simulink model "PVArrayGrid100kw"  (R2019a)
settings: Solver=FixedStepDiscrete  StartTime=0.0  StopTime=2.5  RelTol=1e-3
PreLoadFcn:
  | Ts_Power=1e-6;
  | Ts_Control=100e-6;
InitFcn:
  | Ts_Power=1e-6;
  | Ts_Control=100e-6;
undefined symbols (not defined in the file or in its folder): D1, Delta, DiscIntNeverNeededParam
libraries: powerlib x22, powerlib_meascontrol x11, simulink x2, spsGroundingTransformerLib x1, SignalEditorBlockLib x1, re_lib x1
(part 1 of 2)
settings Model: SimulationMode=accelerator  Creator=The MathWorks, Inc.  LastModifiedBy=HP
settings DataIOCC: LimitDataPoints=on  SaveFormat=Array  SignalLogging=off  DSMLogging=off  ReturnWorkspaceOutputs=off
settings OptimizationCC: ExpressionDepthLimit=2147483647  EfficientMapNaN2IntZero=off  LifeSpan=inf
settings DebuggingCC: UnderspecifiedInitializationDetection=Classic  MergeDetectMultiDrivingBlocksExec=none  SolverPrmCheckMsg=warning  FcnCallInpInsideContextMsg=warning  StateNameClashWarn=warning  SFUnexpectedBacktrackingDiag=warning  SFNoUnconditionalDefaultTransitionDiag=warning  SFExecutionAtInitializationDiag=none  ArithmeticOperatorsInVariantConditions=warning
settings HardwareCC: ProdBitPerPointer=32  ProdBitPerSizeT=32  ProdBitPerPtrDiffT=32  ProdLargestAtomicFloat=None  ProdIntDivRoundTo=Undefined  ProdEndianess=Unspecified  ProdWordSize=32  ProdHWDeviceType=32-bit Generic  TargetBitPerPointer=64  TargetBitPerSizeT=64  TargetBitPerPtrDiffT=64  TargetLongLongMode=on  TargetIntDivRoundTo=Zero  TargetEndianess=LittleEndian  TargetWordSize=64  TargetHWDeviceType=MATLAB Host  ProdEqTarget=off
settings ModelReferenceCC: PropagateSignalLabelsOutOfModel=off
settings SFSimCC: SimUseLocalCustomCode=off
settings CodeAppCC: MaxIdLength=128
settings GRTTargetCC: TargetLangStandard=C89/C90 (ANSI)  CombineOutputUpdateFcns=off  GRTInterface=on
settings ConfigComp: CovMetricSettings=dw  CovSaveCumulativeToWorkspaceVar=on  CovSaveSingleToWorkspaceVar=on  CovExternalEMLEnable=off  CovSFcnEnable=off
settings SimscapeCC: SimscapeNormalizeSystem=off

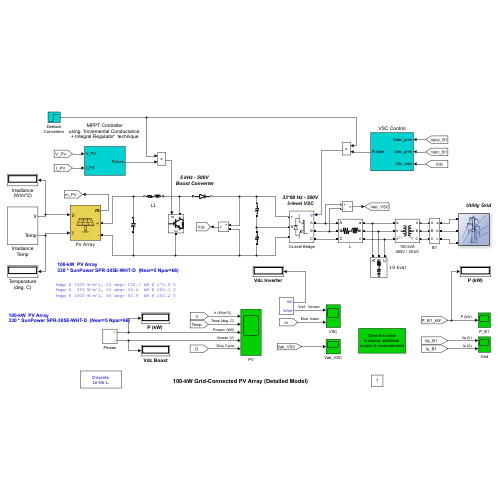
[thumbnail: Simulink's stored preview of the top-level diagram]
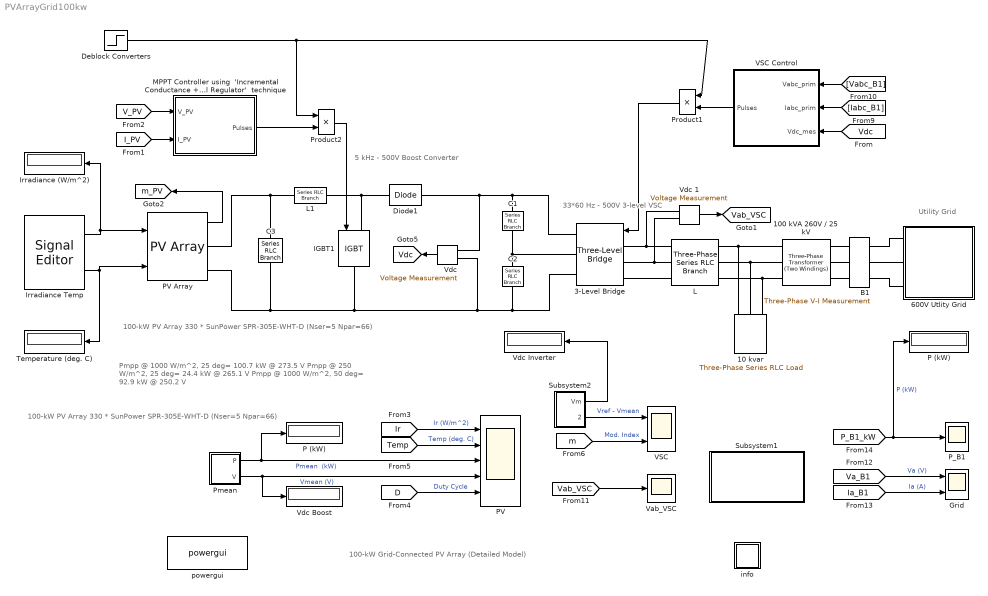
== system PVArrayGrid100kw ==
  note: 5 kHz - 500V
      | Boost Converter
  note: 33*60 Hz - 500V
      | 3-level VSC
  note: 100-kW Grid-Connected PV Array (Detailed Model)
  note: Utility Grid
  note: Pmpp @ 1000 W/m^2, 25 deg= 100.7 kW @ 273.5 V
      | Pmpp @  250 W/m^2, 25 deg= 24.4  kW @ 265.1 V
      | Pmpp @ 1000 W/m^2, 50 deg= 92.9  kW @ 250.2 V
  note: 100-kW  PV Array
      | 330 * SunPower SPR-305E-WHT-D  (Nser=5 Npar=66)
  note: 100-kW  PV Array
      | 330 * SunPower SPR-305E-WHT-D  (Nser=5 Npar=66)
  10 kvar : powerlib/Elements/Three-Phase Series RLC Load  LConnTagsString=A|B|C  Configuration=Y (grounded)  NominalVoltage=240  Vabc=[1e3 1e3 1e3]  Vabcp=[1e3 1e3 1e3]  NominalFrequency=60  UnbalancedPower=off  ActivePower=10e3/100  InductivePower=0  CapacitivePower=10e3  Pabc=[10e3 9e3 11e3]  QLabc=[100 90 110]  QCabc=[100 90 110]  Pabcp=[10e3 9e3 11e3]  QLabcp=[100 90 110]  QCabcp=[100 90 110]  Measurements=None  LoadType=constant Z
  100 kVA 260V / 25 kV : powerlib/Elements/Three-Phase Transformer (Two Windings)  Winding1Connection=Yg  Winding2Connection=Delta (D1)  CoreType=Three single-phase transformers  SetSaturation=off  Hysteresis=off  DataFile='hysteresis'  SetInitialFlux=off  Measurements=None  UNITS=pu  NominalPower=[100e3 , 60 ]  Winding1=[ 25e3 , 0.001 , 0.03 ]  Winding2=[ 260 , 0.001 , 0.03 ]  Rm=500  Lm=500  L0=0.5  Saturation=[ 0,0 ; 0.0024,1.2 ; 1.0,1.52 ]  InitialFluxes=[ 0.8 , -0.8 , 0.7 ]  BreakLoop=off  DiscreteSolver=Trapezoidal iterative  DataType=off  TransfoNumber=0
  3-Level Bridge : powerlib/Power Electronics/Three-Level Bridge  Arms=3  SnubberResistance=1e6  SbubberCapacitance=inf  Device=IGBT / Diodes  Ron=0.2e-3  ForwardVoltages="[  0  0 ]"  Measurements=None
  600V Utlity Grid : Subsystem
      mask Display: image('grid.jpg')
  B1 : powerlib/Measurements/Three-Phase V-I Measurement  VoltageMeasurement=phase-to-ground  SetLabelV=on  LabelV=Vabc_B1  Vpu=off  VpuLL=off  CurrentMeasurement=yes  SetLabelI=on  LabelI=Iabc_B1  Ipu=off  Pbase=100e6  Vbase=500e3  OutputType=Magnitude  PhasorSimulation=off  PSBequivalent=0
  C1 : powerlib/Elements/Series RLC Branch  LConnTagsString=__new0  RConnTagsString=__new0  BranchType=C  Resistance=1.0  Inductance=1.0  SetiL0=off  InitialCurrent=0  Capacitance=12000e-06  Setx0=off  InitialVoltage=0  Measurements=None
  C2 : powerlib/Elements/Series RLC Branch  LConnTagsString=__new0  RConnTagsString=__new0  BranchType=C  Resistance=1.0  Inductance=1.0  SetiL0=off  InitialCurrent=0  Capacitance=12000e-06  Setx0=off  InitialVoltage=0  Measurements=None
  C3 : powerlib/Elements/Series RLC Branch  LConnTagsString=__new0  RConnTagsString=__new0  BranchType=C  Resistance=1.0  Inductance=1.0  SetiL0=off  InitialCurrent=0  Capacitance=100e-6  Setx0=off  InitialVoltage=0  Measurements=Branch voltage
  Deblock Converters : Step  Time=0.05  SampleTime=0
  Diode1 : powerlib/Power Electronics/Diode  Ron=1e-4  Lon=0  Vf=0  IC=0  UseSnubber=off  Rs=inf  Cs=inf  Measurements=off
  Grid : Scope  NumInputPorts=2
  IGBT1 : powerlib/Power Electronics/IGBT  Ron=0.001  Lon=0  Vf=0  Tf=0  Tt=0  IC=0  Rs=1e5  Cs=inf  Measurements=off
  Irradiance (W/m^2) : Display
      settings: Format=bank  Decimation=1000
  Irradiance Temp : SignalEditorBlockLib/Signal Editor  FileName=PVArrayGridData.mat  ActiveScenario=Ramp_up_down_Irradiance  ActiveSignal=Temp  IsBus=off  OutputBusObjectStr=Bus: BusObject  SampleTime=0  OutputAfterFinalValue=Extrapolation  Unit=inherit  PreserveSignalName=on
  L : powerlib/Elements/Three-Phase Series RLC Branch  LConnTagsString=A|B|C  RConnTagsString=A|B|C  BranchType=RL  Resistance=500e-6*377/50/2  Inductance=500e-6/2  Capacitance=inf  Measurements=None
  L1 : powerlib/Elements/Series RLC Branch  LConnTagsString=__new0  RConnTagsString=__new0  BranchType=RL  Resistance=0.005  Inductance=5e-3  SetiL0=off  InitialCurrent=0  Capacitance=1e-6  Setx0=off  InitialVoltage=0  Measurements=None
  "MPPT Controller using  'Incremental Conductance + Integral Regulator'  technique " : Subsystem  mask(Boost Control - MPPT){fc=5000, T_MPPT=200e-6, Dinit=0.5}
      mask prompts: fc "PWM switching frequency (Hz)"; T_MPPT "Time window used by MPPT control (s)"; Dinit "Initial value of duty cycle"
  P (kW) : Display
      settings: Format=bank  Decimation=2000
  "P (kW) " : Display
      settings: Format=bank  Decimation=2000
  PV : Scope  NumInputPorts=5
  PV Array : re_lib/Solar/PV Array  Npar=66  Nser=5  PlotType=array @ 1000 W/m2 & specified temperatures  S_vec="[ 1000  250 ]"  Temp_C_vec="[0 25 50  ]"  ModuleName=SunPower SPR-305E-WHT-D  PlotWhenSelected=off  Pm=305.226  Ncell=96  Voc=64.2  Isc=5.96  Vm=54.7  Im=5.58  beta_Voc_pc=-0.2727  alpha_Isc_pc=0.061745  beta_Voc=-0.17507  alpha_Isc=0.00368  IL=5.9657  I0=6.3076e-12  nI=0.94489  Rsh=393.2054  Rs=0.37428  RobustModel=off  RobustCellTemperature=25  BAL=on  Tc=1e-6  Tfilter=5e-5
  P_B1 : Scope
  Pmean : Subsystem
  Product1 : Product  RndMeth=Zero
  Product2 : Product  RndMeth=Zero
  Subsystem1 : Subsystem
      mask Display: disp('Open this block\nto display additional \nscopes & measurements')
  Subsystem2 : Subsystem
  Temperature (deg. C) : Display
      settings: Format=bank  Decimation=1000
  VSC : Scope  NumInputPorts=2
  VSC Control : Subsystem  mask(VSC Main Controller){nom=[ 100e3  60 ], Vnom=[ 25e3 260 ], Vnom_dc=500, RLxfo=[0.002  0.06 ], RLchoke=[2e-3  250e-6  ], K_VDCreg=[7  800], K_Ireg=[0.3 20], Ts=Ts_Control}
      mask prompts: nom "Nominal power and frequency [ Pnom(VA)  Fnom(Hz) ]:"; Vnom "Nominal primary and secondary voltages (Vrms LL) [ Vnom_prim   Vnom_sec ]:"; Vnom_dc "Nominal DC bus voltage (V):"; RLxfo "Total transformer leakage impedance (pu/Pnom) [ Rxfo  Lxf ]"; RLchoke "Choke impedance [ R(ohm) L(H) ]"; K_VDCreg "VDC regultator gains [ Kp  Ki ]:"; K_Ireg "Current regulator gains [ Kp  Ki ]:"; Ts "Sample time"
      mask init:
      | Pnom=nom(1);
      | Fnom=nom(2);
      | Vnom_prim=Vnom(1);
      | Vnom_sec=Vnom(2);
      | Zbase=Vnom_sec^2/Pnom;
      | Rtot_pu=RLxfo(1) + RLchoke(1)/Zbase;
      | Ltot_pu=RLxfo(2) + RLchoke(2)/(Zbase/(2*pi*Fnom));
      | Kp_VDCreg=K_VDCreg(1);
      | Ki_VDCreg=K_VDCreg(2);
      | Kp_Ireg=K_Ireg(1);
      | Ki_Ireg=K_Ireg(2);
      | Vdc_ref=Vnom_dc;
      | % Used to determine initial value of Boost Control (MPPT)
      | assignin('base','Vdc_ref_Inv',Vdc_ref);
  Vab_VSC : Scope
  "Vdc " : powerlib/Measurements/Voltage Measurement  Tag=PoWeRsYsTeMmEaSuReMeNt  PhasorSimulation=off  OutputType=Magnitude  PSBequivalent=0
  Vdc 1 : powerlib/Measurements/Voltage Measurement  Tag=PoWeRsYsTeMmEaSuReMeNt  PhasorSimulation=off  OutputType=Magnitude  PSBequivalent=0
  Vdc Boost : Display
      settings: Format=bank  Decimation=2000
  Vdc Inverter : Display
      settings: Format=bank  Decimation=2000
  info : Subsystem
      settings: OpenFcn="showExample(\"simscapeelectricalsps/PVArrayGridExample\")"
      mask Display: disp('?')
  powergui : powerlib/powergui  Priority=1  SimulationMode=Discrete  SampleTime=Ts_Power  frequency=60  Iterations=50  frequencyindice=0  Pbase=100e6  ErrMax=1e-4  UnitsV=kV  UnitsW=MW  buscounter=0  FunctionMessages=off  echomessages=off  EnableUseOfTLC=off  CurrentSourceSwitches=off  DisableSnubberDevices=off  DisableRonSwitches=off  DisableVfSwitches=off  DisplayEquations=off  AutomaticDiscreteSolvers=off  SolverType=Tustin/Backward Euler (TBE)  Interpol=off  ExternalGateDelay=off  methode=off  Ts=0  x0status=blocks  SPID=off  SwTol=0  HookPort=off  NonlinearTolerance=1e-8  nMaxIteration=10  ContinueOnMaxIteration=off  RestoreLinks=warning  ResistiveCurrentMeasurement=off  Frange=[0:2:500]  Ylog=off  Xlog=on  ShowGrid=off  save=off  variable=ZData  structure=0  ZoomFFT=on  StartTime=0.0  cycles=1  DisplayStyle=1  fundamental=60  FreqAxis=off  MaxFrequency=1000  frequencyindicesteady=1  RmsSteady=1  display=off
  tag scope: Vab_VSC=global, Vdc=global, m_PV=global
  wires:
  "Vdc "/1 -> [Vdc]
  Product2/1 -> IGBT1/1
  "MPPT Controller using  'Incremental Conductance + Integral Regulator'  technique "/1(Pulses) -> Product2/2
  Deblock Converters/1 -> Product1/1, Product2/1
  [Vabc_B1] -> VSC Control/1(Vabc_prim)
  [Iabc_B1] -> VSC Control/2(Iabc_prim)
  [Vdc] -> VSC Control/3(Vdc_mes)
  VSC Control/1(Pulses) -> Product1/2
  Product1/1 -> 3-Level Bridge/1
  [I_PV] -> "MPPT Controller using  'Incremental Conductance + Integral Regulator'  technique "/2(I_PV)
  [V_PV] -> "MPPT Controller using  'Incremental Conductance + Integral Regulator'  technique "/1(V_PV)
  Pmean/1(P) -> "P (kW) "/1, PV/3  "Pmean  (kW)"
  [m] -> VSC/2  "Mod. Index"
  Vdc 1/1 -> [Vab_VSC]
  [Vab_VSC] -> Vab_VSC/1
  [Ia_B1] -> Grid/2  "Ia (A)"
  [Va_B1] -> Grid/1  "Va (V)"
  [P_B1_kW] -> P_B1/1, P (kW)/1  "P (kW)"
  Pmean/2(V) -> Vdc Boost/1, PV/4  "Vmean (V)"
  Subsystem2/2(VrVm) -> VSC/1  "Vref - Vmean"
  Subsystem2/1(Vm) -> Vdc Inverter/1
  PV Array/1 -> [m_PV]
  Irradiance Temp/1 -> PV Array/1, Irradiance (W/m^2)/1
  Irradiance Temp/2 -> PV Array/2, Temperature (deg. C)/1
  [D] -> PV/5  "Duty Cycle"
  [Temp] -> PV/2  "Temp (deg. C)"
  [Ir] -> PV/1  "Ir (W/m^2)"
  connections:
  3-Level Bridge/RConn1 -- Diode1/RConn1 -- "Vdc "/LConn1 -- C1/LConn1
  L1/RConn1 -- Diode1/LConn1 -- IGBT1/LConn1
  3-Level Bridge/RConn3 -- C2/RConn1 -- "Vdc "/LConn2 -- IGBT1/RConn1 -- PV Array/RConn2 -- C3/RConn1
  3-Level Bridge/LConn1 -- L/LConn1 -- Vdc 1/LConn1
  3-Level Bridge/LConn2 -- L/LConn2 -- Vdc 1/LConn2
  3-Level Bridge/LConn3 -- L/LConn3
  L/RConn1 -- 100 kVA 260V / 25 kV/RConn1 -- 10 kvar/LConn1
  L/RConn2 -- 100 kVA 260V / 25 kV/RConn2 -- 10 kvar/LConn2
  L/RConn3 -- 100 kVA 260V / 25 kV/RConn3 -- 10 kvar/LConn3
  B1/LConn1 -- 100 kVA 260V / 25 kV/LConn1
  B1/LConn2 -- 100 kVA 260V / 25 kV/LConn2
  B1/LConn3 -- 100 kVA 260V / 25 kV/LConn3
  C2/LConn1 -- C1/RConn1 -- 3-Level Bridge/RConn2
  C3/LConn1 -- PV Array/RConn1 -- L1/LConn1
  B1/RConn2 -- 600V Utlity Grid/LConn2
  B1/RConn1 -- 600V Utlity Grid/LConn1
  B1/RConn3 -- 600V Utlity Grid/LConn3

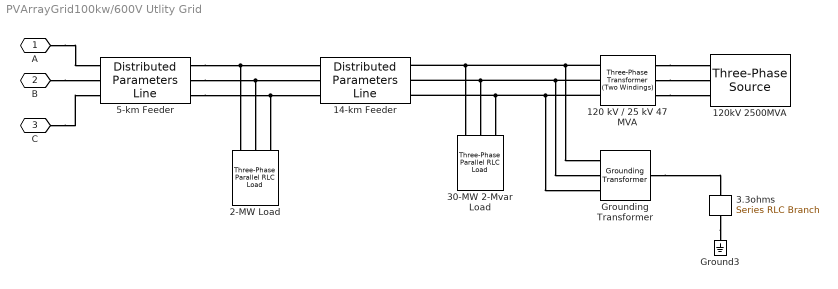
== system PVArrayGrid100kw/600V Utlity Grid ==
  120 kV / 25 kV 47 MVA : powerlib/Elements/Three-Phase Transformer (Two Windings)  Winding1Connection=Yg  Winding2Connection=Delta (D1)  CoreType=Three single-phase transformers  SetSaturation=off  Hysteresis=off  DataFile='basic_model'  SetInitialFlux=off  Measurements=None  UNITS=pu  NominalPower=[47e6 60 ]  Winding1="[ 120e3  0.08/30   0.08 ]"  Winding2="[ 25e3  0.08/30  0.08]"  Rm=500  Lm=500  L0=0.5  Saturation="[ 0,0  ;  0.005,1.2  ;  1.0,1.4 ]"  InitialFluxes=[ 0.8 , -0.8 , 0.7 ]  BreakLoop=off  DiscreteSolver=Trapezoidal iterative  DataType=off  TransfoNumber=0
  120kV 2500MVA : powerlib/Electrical Sources/Three-Phase Source  InternalConnection=Yg  VoltagePhases=off  Voltage=120e3  PhaseAngle=0  Voltage_phases=[25e3 25e3 25e3]/sqrt(3)  PhaseAngles_phases=[0 -120 +120]  Frequency=60  NonIdealSource=on  SpecifyImpedance=on  Resistance=0.8929  Inductance=16.58e-3  ShortCircuitLevel=2500e6  BaseVoltage=120e3  XRratio=7  BusType=swing  Pref=0  Qref=0  Prefabc=[10e3, 10e3, 10e3]  Qrefabc=[0, 0, 0]  Qmin=-inf  Qmax=inf
  14-km Feeder : powerlib/Elements/Distributed Parameters Line  Phases=3  Length=14  Frequency=60  Resistance=[0.1153 0.413]  Inductance=[1.05e-3 3.32e-3]  Capacitance=[11.33e-009 5.01e-009]  x1=[-5.8e-05 -3.04262372149305e-09 0 0;-5.7e-05 -3.04220635150541e-09 0 0;-5.6e-05 -3.0417885491524e-09 0 0;-5.5e-05 -3.04137031449339e-09 0 0;-5.4e-05 -3.04095164758784e-09 0 0;-5.3e-05 -3.04053254849524e-09 0 0;-5.2e-05 -3.04011301727516e-09 0 0;-5.1e-05 -3.03969305398722e-09 0 0;-5e-05 -3.0392726586911e-09 0 0;-4.9e-05 -3.03885183144656e-09 -3790.73535189758 -24061.413420025;-4.8e-05 -3.0384305723134e-09 -3781.66414358218 -24062.8407837194;-4.7e-05 -3.0380088813515e-09 -3772.59239780798 -24064.2647275475;-4.6e-05 -3.03758675862078e-09 -3763.52011586425 -24065.6852513069;-4.5e-05 -3.03716420418123e-09 -3754.44729904039 -24067.1023547957;-4.4e-05 -3.03674121809293e-09 -3745.37394862584 -24068.5160378125;-4.3e-05 -3.03631780041596e-09 -3736.30006591012 -24069.9263001565;-4.2e-05 -3.03589395121053e-09 -3727.22565218283 -24071.3331416271;-4.1e-05 -3.03546967053686e-09 -3718.15070873366 -24072.7365620244;-4e-05 -3.03504495845525e-09 -3709.07523685234 -24074.136561149;-3.9e-05 -3.03461981502607e-09 -3699.99923782872 -24075.5331388019;-3.8e-05 -3.03419424030973e-09 -3690.92271295269 -24076.9262947847;-3.7e-05 -3.03376823436673e-09 -3681.84566351423 -24078.3160288992;-3.6e-05 -3.0333417972576e-09 -3672.76809080339 -24079.7023409481;-3.5e-05 -3.03291492904295e-09 -3663.6899961103 -24081.0852307342;-3.4e-05 -3.03248762978346e-09 -3654.61138072515 -24082.4646980611;-3.3e-05 -3.03205989953984e-09 -3645.53224593822 -24083.8407427326;-3.2e-05 -3.03163173837289e-09 -3636.45259303985 -24085.2133645533;-3.1e-05 -3.03120314634346e-09 -3627.37242332047 -24086.582563328;-3e-05 -3.03077412351246e-09 -3618.29173807058 -24087.9483388622;-2.9e-05 -3.03034466994086e-09 -3609.21053858073 -24089.3106909617;-2.8e-05 -3.02991478568971e-09 -3600.12882614158 -24090.6696194329;-2.7e-05 -3.02948447082009e-09 -3591.04660204383 -24092.0251240827;-2.6e-05 -3.02905372539317e-09 -3581.96386757827 -24093.3772047185;-2.5e-05 -3.02862254947016e-09 -3572.88062403576 -24094.725861148;-2.4e-05 -3.02819094311234e-09 -3563.79687270724 -24096.0710931796;-2.3e-05 -3.02775890638106e-09 -3554.7126148837 -24097.4129006222;-2.2e-05 -3.02732643933771e-09 -3545.62785185622 -24098.7512832849;-2.1e-05 -3.02689354204376e-09 -3536.54258491595 -24100.0862409777;-2e-05 -3.02646021456073e-09 -3527.4568153541 -24101.4177735107;-1.9e-05 -3.02602645695021e-09 -3518.37054446198 -24102.7458806947;-1.8e-05 -3.02559226927385e-09 -3509.28377353094 -24104.0705623411;-1.7e-05 -3.02515765159334e-09 -3500.19650385241 -24105.3918182614;-1.6e-05 -3.02472260397047e-09 -3491.10873671789 -24106.709648268;-1.5e-05 -3.02428712646707e-09 -3482.02047341897 -24108.0240521735;-1.4e-05 -3.02385121914501e-09 -3472.93171524728 -24109.3350297912;-1.3e-05 -3.02341488206626e-09 -3463.84246349454 -24110.6425809346;-1.2e-05 -3.02297811529282e-09 -3454.75271945254 -24111.9467054181;-1.1e-05 -3.02254091888678e-09 -3445.66248441313 -24113.2474030561;-1e-05 -3.02210329291027e-09 -3436.57175966824 -24114.544673664;-9e-06 -3.02166523742548e-09 -3427.48054650986 -24115.8385170573;-8e-06 -3.02122675249467e-09 -3418.38884623006 -24117.128933052;-7e-06 -3.02078783818016e-09 -3409.29666012096 -24118.4159214649;-6e-06 -3.02034849454434e-09 -3400.20398947478 -24119.6994821131;-5e-06 -3.01990872164963e-09 -3391.11083558378 -24120.979614814;-4e-06 -3.01946851955854e-09 -3382.0171997403 -24122.2563193858;-3e-06 -3.01902788833364e-09 -3372.92308323675 -24123.529595647;-2e-06 -3.01858682803754e-09 -3363.82848736561 -24124.7994434166;-1e-06 -3.01814533873294e-09 -3354.73341341942 -24126.0658625142]  x2=[-5.8e-05 -3.19786387480592e-09 0 0;-5.7e-05 -3.19737360997783e-09 0 0;-5.6e-05 -3.19688289073164e-09 0 0;-5.5e-05 -3.1963917171371e-09 0 0;-5.4e-05 -3.19590008926401e-09 0 0;-5.3e-05 -3.19540800718224e-09 0 0;-5.2e-05 -3.19491547096173e-09 0 0;-5.1e-05 -3.19442248067248e-09 0 0;-5e-05 -3.19392903638456e-09 0 0;-4.9e-05 -3.19343513816809e-09 -3379.39242591108 -24244.0512732151;-4.8e-05 -3.19294078609326e-09 -3370.25239397928 -24245.323551305;-4.7e-05 -3.19244598023035e-09 -3361.11188305944 -24246.5923835937;-4.6e-05 -3.19195072064966e-09 -3351.97089445066 -24247.8577699009;-4.5e-05 -3.19145500742159e-09 -3342.82942945205 -24249.1197100467;-4.4e-05 -3.19095884061659e-09 -3333.68748936283 -24250.3782038519;-4.3e-05 -3.19046222030517e-09 -3324.54507548227 -24251.6332511374;-4.2e-05 -3.18996514655792e-09 -3315.40218910971 -24252.884851725;-4.1e-05 -3.18946761944548e-09 -3306.25883154457 -24254.1330054368;-4e-05 -3.18896963903856e-09 -3297.1150040863 -24255.3777120954;-3.9e-05 -3.18847120540794e-09 -3287.97070803447 -24256.6189715239;-3.8e-05 -3.18797231862445e-09 -3278.82594468867 -24257.8567835459;-3.7e-05 -3.18747297875899e-09 -3269.68071534858 -24259.0911479854;-3.6e-05 -3.18697318588254e-09 -3260.53502131394 -24260.3220646671;-3.5e-05 -3.18647294006612e-09 -3251.38886388456 -24261.5495334159;-3.4e-05 -3.18597224138084e-09 -3242.24224436031 -24262.7735540575;-3.3e-05 -3.18547108989785e-09 -3233.09516404113 -24263.9941264179;-3.2e-05 -3.18496948568837e-09 -3223.94762422702 -24265.2112503236;-3.1e-05 -3.1844674288237e-09 -3214.79962621805 -24266.4249256016;-3e-05 -3.18396491937519e-09 -3205.65117131437 -24267.6351520794;-2.9e-05 -3.18346195741426e-09 -3196.50226081616 -24268.841929585;-2.8e-05 -3.18295854301239e-09 -3187.35289602369 -24270.045257947;-2.7e-05 -3.18245467624112e-09 -3178.20307823729 -24271.2451369943;-2.6e-05 -3.18195035717207e-09 -3169.05280875736 -24272.4415665564;-2.5e-05 -3.18144558587691e-09 -3159.90208888434 -24273.6345464632;-2.4e-05 -3.18094036242738e-09 -3150.75091991877 -24274.8240765452;-2.3e-05 -3.18043468689528e-09 -3141.59930316123 -24276.0101566333;-2.2e-05 -3.17992855935249e-09 -3132.44723991236 -24277.192786559;-2.1e-05 -3.17942197987093e-09 -3123.29473147288 -24278.3719661542;-2e-05 -3.1789149485226e-09 -3114.14177914356 -24279.5476952513;-1.9e-05 -3.17840746537956e-09 -3104.98838422525 -24280.7199736831;-1.8e-05 -3.17789953051394e-09 -3095.83454801884 -24281.8888012832;-1.7e-05 -3.17739114399792e-09 -3086.68027182529 -24283.0541778853;-1.6e-05 -3.17688230590375e-09 -3077.52555694565 -24284.2161033239;-1.5e-05 -3.17637301630377e-09 -3068.37040468099 -24285.3745774338;-1.4e-05 -3.17586327527034e-09 -3059.21481633246 -24286.5296000503;-1.3e-05 -3.17535308287591e-09 -3050.05879320128 -24287.6811710094;-1.2e-05 -3.17484243919299e-09 -3040.90233658873 -24288.8292901473;-1.1e-05 -3.17433134429415e-09 -3031.74544779614 -24289.9739573009;-1e-05 -3.17381979825204e-09 -3022.5881281249 -24291.1151723075;-9e-06 -3.17330780113935e-09 -3013.43037887649 -24292.2529350049;-8e-06 -3.17279535302886e-09 -3004.27220135241 -24293.3872452314;-7e-06 -3.17228245399339e-09 -2995.11359685425 -24294.5181028257;-6e-06 -3.17176910410583e-09 -2985.95456668366 -24295.6455076273;-5e-06 -3.17125530343915e-09 -2976.79511214232 -24296.7694594758;-4e-06 -3.17074105206636e-09 -2967.63523453202 -24297.8899582115;-3e-06 -3.17022635006056e-09 -2958.47493515457 -24299.0070036751;-2e-06 -3.16971119749489e-09 -2949.31421531184 -24300.1205957079;-1e-06 -3.16919559444257e-09 -2940.1530763058 -24301.2307341517]  x3=[-5.8e-05 -1.60560160529195e-11 0 0;-5.7e-05 -1.60568474458934e-11 0 0;-5.6e-05 -1.60576765568311e-11 0 0;-5.5e-05 -1.6058503385615e-11 0 0;-5.4e-05 -1.60593279321273e-11 0 0;-5.3e-05 -1.60601501962511e-11 0 0;-5.2e-05 -1.60609701778693e-11 0 0;-5.1e-05 -1.60617878768654e-11 0 0;-5e-05 -1.60626032931233e-11 0 0;-4.9e-05 -1.60634164265271e-11 -23.5442847382492 -155.681477773822;-4.8e-05 -1.60642272769611e-11 -23.4855925321305 -155.690342696943;-4.7e-05 -1.60650358443102e-11 -23.4268969881853 -155.699185492994;-4.6e-05 -1.60658421284594e-11 -23.3681981147557 -155.708006160718;-4.5e-05 -1.60666461292941e-11 -23.3094959201839 -155.716804698862;-4.4e-05 -1.60674478467001e-11 -23.2507904128129 -155.725581106176;-4.3e-05 -1.60682472805634e-11 -23.1920816009861 -155.734335381411;-4.2e-05 -1.60690444307705e-11 -23.1333694930472 -155.743067523325;-4.1e-05 -1.6069839297208e-11 -23.0746540973407 -155.751777530675;-4e-05 -1.60706318797629e-11 -23.0159354222111 -155.760465402224;-3.9e-05 -1.60714221783226e-11 -22.9572134760039 -155.769131136737;-3.8e-05 -1.60722101927748e-11 -22.8984882670646 -155.777774732983;-3.7e-05 -1.60729959230076e-11 -22.8397598037395 -155.786396189732;-3.6e-05 -1.60737793689091e-11 -22.7810280943752 -155.794995505761;-3.5e-05 -1.60745605303681e-11 -22.7222931473187 -155.803572679846;-3.4e-05 -1.60753394072736e-11 -22.6635549709176 -155.812127710769;-3.3e-05 -1.60761159995148e-11 -22.6048135735199 -155.820660597314;-3.2e-05 -1.60768903069815e-11 -22.5460689634741 -155.829171338267;-3.1e-05 -1.60776623295634e-11 -22.487321149129 -155.83765993242;-3e-05 -1.6078432067151e-11 -22.4285701388341 -155.846126378567;-2.9e-05 -1.60791995196349e-11 -22.3698159409392 -155.854570675503;-2.8e-05 -1.60799646869058e-11 -22.3110585637946 -155.862992822028;-2.7e-05 -1.60807275688552e-11 -22.252298015751 -155.871392816947;-2.6e-05 -1.60814881653746e-11 -22.1935343051596 -155.879770659064;-2.5e-05 -1.60822464763559e-11 -22.134767440372 -155.88812634719;-2.4e-05 -1.60830025016912e-11 -22.0759974297402 -155.896459880136;-2.3e-05 -1.60837562412733e-11 -22.017224281617 -155.904771256719;-2.2e-05 -1.60845076949949e-11 -21.9584480043551 -155.913060475756;-2.1e-05 -1.60852568627492e-11 -21.8996686063081 -155.921327536071;-2e-05 -1.60860037444298e-11 -21.8408860958297 -155.929572436487;-1.9e-05 -1.60867483399305e-11 -21.7821004812744 -155.937795175834;-1.8e-05 -1.60874906491456e-11 -21.7233117709968 -155.945995752943;-1.7e-05 -1.60882306719694e-11 -21.6645199733521 -155.954174166647;-1.6e-05 -1.60889684082968e-11 -21.605725096696 -155.962330415786;-1.5e-05 -1.60897038580231e-11 -21.5469271493845 -155.970464499199;-1.4e-05 -1.60904370210435e-11 -21.4881261397741 -155.978576415731;-1.3e-05 -1.60911678972541e-11 -21.4293220762218 -155.986666164228;-1.2e-05 -1.60918964865508e-11 -21.3705149670848 -155.994733743541;-1.1e-05 -1.60926227888302e-11 -21.3117048207212 -156.002779152524;-1e-05 -1.60933468039889e-11 -21.2528916454889 -156.010802390033;-9e-06 -1.60940685319242e-11 -21.1940754497468 -156.018803454927;-8e-06 -1.60947879725334e-11 -21.135256241854 -156.02678234607;-7e-06 -1.60955051257143e-11 -21.0764340301698 -156.034739062328;-6e-06 -1.6096219991365e-11 -21.0176088230543 -156.042673602569;-5e-06 -1.60969325693838e-11 -20.9587806288679 -156.050585965666;-4e-06 -1.60976428596695e-11 -20.8999494559714 -156.058476150495;-3e-06 -1.60983508621212e-11 -20.8411153127259 -156.066344155934;-2e-06 -1.60990565766382e-11 -20.7822782074932 -156.074189980865;-1e-06 -1.60997600031202e-11 -20.7234381486352 -156.082013624173]  x4=[-5.8e-05 7.96597166434352e-12 0 0;-5.7e-05 7.96849067585659e-12 0 0;-5.6e-05 7.97100855486942e-12 0 0;-5.5e-05 7.97352530102418e-12 0 0;-5.4e-05 7.97604091396316e-12 0 0;-5.3e-05 7.97855539332885e-12 0 0;-5.2e-05 7.98106873876388e-12 0 0;-5.1e-05 7.98358094991106e-12 0 0;-5e-05 7.98609202641334e-12 0 0;-4.9e-05 7.98860196791383e-12 -1.35581366009424 -2.15298522698338;-4.8e-05 7.99111077405583e-12 -1.3550019074591 -2.15349620368578;-4.7e-05 7.99361844448276e-12 -1.35418996224797 -2.15400687432833;-4.6e-05 7.99612497883825e-12 -1.35337782457625 -2.15451723883847;-4.5e-05 7.99863037676605e-12 -1.35256549455936 -2.15502729714366;-4.4e-05 8.0011346379101e-12 -1.35175297231274 -2.15553704917141;-4.3e-05 8.00363776191446e-12 -1.35094025795188 -2.15604649484927;-4.2e-05 8.00613974842341e-12 -1.35012735159228 -2.15655563410485;-4.1e-05 8.00864059708135e-12 -1.34931425334948 -2.15706446686577;-4e-05 8.01114030753286e-12 -1.34850096333903 -2.15757299305973;-3.9e-05 8.01363887942267e-12 -1.34768748167652 -2.15808121261444;-3.8e-05 8.01613631239567e-12 -1.34687380847756 -2.15858912545769;-3.7e-05 8.01863260609693e-12 -1.34605994385779 -2.15909673151728;-3.6e-05 8.02112776017167e-12 -1.34524588793289 -2.15960403072108;-3.5e-05 8.02362177426527e-12 -1.34443164081854 -2.16011102299698;-3.4e-05 8.02611464802327e-12 -1.34361720263048 -2.16061770827293;-3.3e-05 8.02860638109139e-12 -1.34280257348445 -2.16112408647691;-3.2e-05 8.03109697311548e-12 -1.34198775349622 -2.16163015753697;-3.1e-05 8.0335864237416e-12 -1.34117274278161 -2.16213592138118;-3e-05 8.03607473261591e-12 -1.34035754145644 -2.16264137793765;-2.9e-05 8.03856189938479e-12 -1.33954214963657 -2.16314652713455;-2.8e-05 8.04104792369475e-12 -1.33872656743788 -2.16365136890008;-2.7e-05 8.04353280519248e-12 -1.3379107949763 -2.16415590316251;-2.6e-05 8.0460165435248e-12 -1.33709483236775 -2.16466012985012;-2.5e-05 8.04849913833874e-12 -1.33627867972821 -2.16516404889124;-2.4e-05 8.05098058928145e-12 -1.33546233717367 -2.16566766021427;-2.3e-05 8.05346089600027e-12 -1.33464580482014 -2.16617096374763;-2.2e-05 8.05594005814269e-12 -1.33382908278368 -2.16667395941978;-2.1e-05 8.05841807535637e-12 -1.33301217118037 -2.16717664715924;-2e-05 8.06089494728912e-12 -1.33219507012629 -2.16767902689457;-1.9e-05 8.06337067358893e-12 -1.33137777973759 -2.16818109855437;-1.8e-05 8.06584525390394e-12 -1.33056030013041 -2.16868286206727;-1.7e-05 8.06831868788246e-12 -1.32974263142094 -2.16918431736198;-1.6e-05 8.07079097517295e-12 -1.32892477372538 -2.16968546436722;-1.5e-05 8.07326211542406e-12 -1.32810672715998 -2.17018630301177;-1.4e-05 8.07573210828457e-12 -1.32728849184099 -2.17068683322444;-1.3e-05 8.07820095340344e-12 -1.32647006788471 -2.17118705493411;-1.2e-05 8.08066865042981e-12 -1.32565145540744 -2.17168696806968;-1.1e-05 8.08313519901294e-12 -1.32483265452554 -2.17218657256009;-1e-05 8.0856005988023e-12 -1.32401366535538 -2.17268586833435;-9e-06 8.08806484944748e-12 -1.32319448801335 -2.17318485532149;-8e-06 8.09052795059828e-12 -1.32237512261586 -2.1736835334506;-7e-06 8.09298990190462e-12 -1.32155556927939 -2.1741819026508;-6e-06 8.09545070301661e-12 -1.32073582812039 -2.17467996285127;-5e-06 8.09791035358451e-12 -1.31991589925538 -2.17517771398121;-4e-06 8.10036885325875e-12 -1.31909578280088 -2.17567515596989;-3e-06 8.10282620168993e-12 -1.31827547887346 -2.17617228874661;-2e-06 8.1052823985288e-12 -1.31745498758968 -2.17666911224072;-1e-06 8.10773744342627e-12 -1.31663430906618 -2.1771656263816]  x5=5.70973484498186e-05  V1=[0 0 0 2.868e-09 2.436e+04 2.436e+04;0 0 0 377 377 377;1.571 1.571 1.571 -0.5389 -0.156 -1.727]  V2=[0 0 0 2.996e-09 2.448e+04 2.448e+04;0 0 0 377 377 377;1.571 1.571 1.571 -0.5232 -0.1382 -1.709]  I1=[0 0 0 1.022e-11 157.5 157.5;0 0 0 377 377 377;1.571 1.571 1.571 -1.198 -0.1498 -1.721]  I2=[0 0 0 6.231e-12 2.544 2.544;0 0 0 377 377 377;1.571 1.571 1.571 1.184 -0.5617 -2.133]  nHarmo=2  Measurements=None  Decoupling=off  VsMag0=0  VrMag0=0  VsAngle0=0  VrAngle0=0  IsMag0=0  IrMag0=0  IsAngle0=0  IrAngle0=0
  2-MW Load : powerlib/Elements/Three-Phase Parallel RLC Load  LConnTagsString=A|B|C  Configuration=Y (grounded)  NominalVoltage=25e3  Vabc=[1e3 1e3 1e3]  Vabcp=[1e3 1e3 1e3]  NominalFrequency=60  UnbalancedPower=off  ActivePower=2e6  InductivePower=0  CapacitivePower=0  Pabc=[10e3 9e3 11e3]  QLabc=[100 90 110]  QCabc=[100 90 110]  Pabcp=[10e3 9e3 11e3]  QLabcp=[100 90 110]  QCabcp=[100 90 110]  Measurements=None  LoadType=constant Z
  "3.3ohms " : powerlib/Elements/Series RLC Branch  LConnTagsString=__new0  RConnTagsString=__new0  BranchType=R  Resistance=3.3  Inductance=[]  SetiL0=off  InitialCurrent=0  Capacitance=[]  Setx0=off  InitialVoltage=0  Measurements=None
  30-MW 2-Mvar Load : powerlib/Elements/Three-Phase Parallel RLC Load  LConnTagsString=A|B|C  Configuration=Y (grounded)  NominalVoltage=25e3  Vabc=[1e3 1e3 1e3]  Vabcp=[1e3 1e3 1e3]  NominalFrequency=60  UnbalancedPower=off  ActivePower=30e6  InductivePower=2e6  CapacitivePower=0  Pabc=[10e3 9e3 11e3]  QLabc=[100 90 110]  QCabc=[100 90 110]  Pabcp=[10e3 9e3 11e3]  QLabcp=[100 90 110]  QCabcp=[100 90 110]  Measurements=None  LoadType=constant Z
  5-km Feeder : powerlib/Elements/Distributed Parameters Line  Phases=3  Length=5  Frequency=60  Resistance=[0.1153 0.413]  Inductance=[1.05e-3 3.32e-3]  Capacitance=[11.33e-009 5.01e-009]  x1=[-2.1e-05 -2.98680502698762e-09 -3537.17773129419 -24101.4118174689;-2e-05 -2.98637501152554e-09 -3528.09146195667 -24102.7435893523;-1.9e-05 -2.98594457163296e-09 -3519.00469119866 -24104.0719356983;-1.8e-05 -2.98551370737107e-09 -3509.9174203116 -24105.396856318;-1.7e-05 -2.9850824188011e-09 -3500.82965058701 -24106.7183510233;-1.6e-05 -2.98465070598435e-09 -3491.74138331644 -24108.0364196263;-1.5e-05 -2.98421856898217e-09 -3482.65261979156 -24109.3510619397;-1.4e-05 -2.98378600785597e-09 -3473.56336130406 -24110.6622777766;-1.3e-05 -2.98335302266725e-09 -3464.47360914575 -24111.9700669507;-1.2e-05 -2.98291961347752e-09 -3455.38336460847 -24113.2744292761;-1.1e-05 -2.98248578034839e-09 -3446.29262898416 -24114.5753645675;-1e-05 -2.98205152334152e-09 -3437.20140356481 -24115.8728726399;-9e-06 -2.98161684251862e-09 -3428.10968964248 -24117.1669533089;-8e-06 -2.98118173794147e-09 -3419.01748850931 -24118.4576063906;-7e-06 -2.98074620967192e-09 -3409.9248014575 -24119.7448317017;-6e-06 -2.98031025777185e-09 -3400.83162977934 -24121.0286290591;-5e-06 -2.97987388230322e-09 -3391.73797476716 -24122.3089982804;-4e-06 -2.97943708332807e-09 -3382.64383771336 -24123.5859391836;-3e-06 -2.97899986090845e-09 -3373.54921991044 -24124.8594515872;-2e-06 -2.97856221510652e-09 -3364.45412265094 -24126.1295353103;-1e-06 -2.97812414598447e-09 -3355.35854722748 -24127.3961901723]  x2=[-2.1e-05 -3.02689354204376e-09 -3536.54258491595 -24100.0862409777;-2e-05 -3.02646021456073e-09 -3527.4568153541 -24101.4177735107;-1.9e-05 -3.02602645695021e-09 -3518.37054446198 -24102.7458806947;-1.8e-05 -3.02559226927385e-09 -3509.28377353094 -24104.0705623411;-1.7e-05 -3.02515765159334e-09 -3500.19650385241 -24105.3918182614;-1.6e-05 -3.02472260397047e-09 -3491.10873671789 -24106.709648268;-1.5e-05 -3.02428712646707e-09 -3482.02047341897 -24108.0240521735;-1.4e-05 -3.02385121914501e-09 -3472.93171524728 -24109.3350297912;-1.3e-05 -3.02341488206626e-09 -3463.84246349454 -24110.6425809346;-1.2e-05 -3.02297811529282e-09 -3454.75271945254 -24111.9467054181;-1.1e-05 -3.02254091888678e-09 -3445.66248441313 -24113.2474030561;-1e-05 -3.02210329291027e-09 -3436.57175966824 -24114.544673664;-9e-06 -3.02166523742548e-09 -3427.48054650986 -24115.8385170573;-8e-06 -3.02122675249467e-09 -3418.38884623006 -24117.128933052;-7e-06 -3.02078783818016e-09 -3409.29666012096 -24118.4159214649;-6e-06 -3.02034849454434e-09 -3400.20398947478 -24119.6994821131;-5e-06 -3.01990872164963e-09 -3391.11083558378 -24120.979614814;-4e-06 -3.01946851955854e-09 -3382.0171997403 -24122.2563193858;-3e-06 -3.01902788833364e-09 -3372.92308323675 -24123.529595647;-2e-06 -3.01858682803754e-09 -3363.82848736561 -24124.7994434166;-1e-06 -3.01814533873294e-09 -3354.73341341942 -24126.0658625142]  x3=[-2.1e-05 -8.69366441932856e-12 -11.1569792961313 -79.1361755515038;-2e-05 -8.69500235302852e-12 -11.1271448686807 -79.1403760099997;-1.9e-05 -8.69633905097472e-12 -11.0973088598146 -79.1445652208831;-1.8e-05 -8.69767451297721e-12 -11.0674712737735 -79.1487431835587;-1.7e-05 -8.69900873884617e-12 -11.0376321147979 -79.1529098974328;-1.6e-05 -8.70034172839199e-12 -11.0077913871286 -79.1570653619132;-1.5e-05 -8.70167348142522e-12 -10.9779490950066 -79.1612095764092;-1.4e-05 -8.70300399775658e-12 -10.9481052426733 -79.1653425403319;-1.3e-05 -8.70433327719698e-12 -10.91825983437 -79.169464253094;-1.2e-05 -8.70566131955751e-12 -10.8884128743385 -79.1735747141095;-1.1e-05 -8.70698812464941e-12 -10.8585643668207 -79.1776739227944;-1e-05 -8.70831369228411e-12 -10.8287143160588 -79.181761878566;-9e-06 -8.70963802227323e-12 -10.798862726295 -79.1858385808433;-8e-06 -8.71096111442855e-12 -10.7690096017721 -79.189904029047;-7e-06 -8.71228296856202e-12 -10.7391549467327 -79.1939582225993;-6e-06 -8.71360358448579e-12 -10.7092987654198 -79.198001160924;-5e-06 -8.71492296201216e-12 -10.6794410620768 -79.2020328434464;-4e-06 -8.71624110095362e-12 -10.6495818409471 -79.2060532695937;-3e-06 -8.71755800112283e-12 -10.6197211062742 -79.2100624387943;-2e-06 -8.71887366233263e-12 -10.5898588623022 -79.2140603504786;-1e-06 -8.72018808439604e-12 -10.559995113275 -79.2180470040782]  x4=[-2.1e-05 -1.44476194922777e-12 -12.5606324025929 -78.9000787577064;-2e-05 -1.44169215687708e-12 -12.5308868817893 -78.9048083977215;-1.9e-05 -1.43862215962977e-12 -12.5011395800673 -78.9095268236036;-1.8e-05 -1.43555195792217e-12 -12.4713905016545 -78.9142340346822;-1.7e-05 -1.43248155219063e-12 -12.441639650779 -78.9189300302881;-1.6e-05 -1.42941094287151e-12 -12.411887031669 -78.9236148097541;-1.5e-05 -1.42634013040121e-12 -12.382132648553 -78.9282883724143;-1.4e-05 -1.42326911521618e-12 -12.3523765056599 -78.9329507176044;-1.3e-05 -1.42019789775286e-12 -12.3226186072186 -78.937601844662;-1.2e-05 -1.41712647844775e-12 -12.2928589574584 -78.9422417529258;-1.1e-05 -1.41405485773736e-12 -12.2630975606087 -78.9468704417366;-1e-05 -1.41098303605824e-12 -12.2333344208994 -78.9514879104364;-9e-06 -1.40791101384696e-12 -12.2035695425605 -78.9560941583691;-8e-06 -1.40483879154013e-12 -12.1738029298222 -78.9606891848799;-7e-06 -1.40176636957437e-12 -12.144034586915 -78.9652729893158;-6e-06 -1.39869374838636e-12 -12.1142645180696 -78.9698455710254;-5e-06 -1.39562092841277e-12 -12.0844927275171 -78.9744069293587;-4e-06 -1.39254791009031e-12 -12.0547192194886 -78.9789570636676;-3e-06 -1.38947469385575e-12 -12.0249439982158 -78.9834959733053;-2e-06 -1.38640128014584e-12 -11.9951670679301 -78.9880236576267;-1e-06 -1.3833276693974e-12 -11.9653884328638 -78.9925401159885]  x5=2.03919101606495e-05  V1=[0 0 0 2.827e-09 2.436e+04 2.436e+04;0 0 0 377 377 377;1.571 1.571 1.571 -0.5179 -0.1443 -1.715]  V2=[0 0 0 2.868e-09 2.436e+04 2.436e+04;0 0 0 377 377 377;1.571 1.571 1.571 -0.5251 -0.1443 -1.715]  I1=[0 0 0 7.018e-12 79.92 79.92;0 0 0 377 377 377;1.571 1.571 1.571 -1.622 -0.1386 -1.709]  I2=[0 0 0 7.946e-12 79.89 79.89;0 0 0 377 377 377;1.571 1.571 1.571 0.3547 -0.1565 -1.727]  nHarmo=2  Measurements=None  Decoupling=off  VsMag0=0  VrMag0=0  VsAngle0=0  VrAngle0=0  IsMag0=0  IrMag0=0  IsAngle0=0  IrAngle0=0
  Ground3 : powerlib/Elements/Ground  LConnTagsString=a
  "Grounding Transformer " : spsGroundingTransformerLib/Grounding Transformer   UNITS=pu  NominalPower="[100e6   60]"  NominalVoltage=25e3  ZeroSequenceImpedance_pu=[0.025 0.75]  MagnetizationBranch_pu=[500 500]  ZeroSequenceImpedance_SI=[0.052083 589.05]  MagnetizationBranch_SI=[1041.7 3.927e+005]  Measurements=None
  A : PMIOPort  Side=Left
  B : PMIOPort  Port=2  Side=Left
  C : PMIOPort  Port=3  Side=Left
  connections:
  "3.3ohms "/RConn1 -- Ground3/LConn1
  120 kV / 25 kV 47 MVA/LConn1 -- 120kV 2500MVA/RConn1
  120 kV / 25 kV 47 MVA/LConn2 -- 120kV 2500MVA/RConn2
  120 kV / 25 kV 47 MVA/LConn3 -- 120kV 2500MVA/RConn3
  120 kV / 25 kV 47 MVA/RConn1 -- "Grounding Transformer "/LConn1 -- 14-km Feeder/RConn1 -- 30-MW 2-Mvar Load/LConn1
  120 kV / 25 kV 47 MVA/RConn2 -- "Grounding Transformer "/LConn2 -- 14-km Feeder/RConn2 -- 30-MW 2-Mvar Load/LConn2
  120 kV / 25 kV 47 MVA/RConn3 -- "Grounding Transformer "/LConn3 -- 14-km Feeder/RConn3 -- 30-MW 2-Mvar Load/LConn3
  5-km Feeder/RConn1 -- 14-km Feeder/LConn1 -- 2-MW Load/LConn1
  5-km Feeder/RConn2 -- 14-km Feeder/LConn2 -- 2-MW Load/LConn2
  5-km Feeder/RConn3 -- 14-km Feeder/LConn3 -- 2-MW Load/LConn3
  A/RConn1 -- 5-km Feeder/LConn1
  B/RConn1 -- 5-km Feeder/LConn2
  C/RConn1 -- 5-km Feeder/LConn3
  "Grounding Transformer "/RConn1 -- "3.3ohms "/LConn1

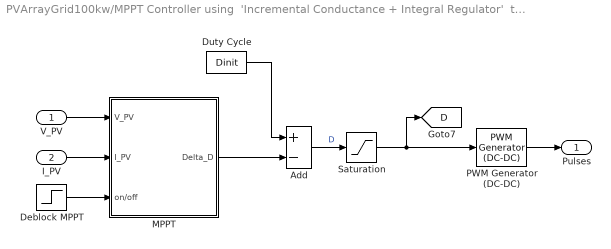
== system PVArrayGrid100kw/MPPT Controller using  'Incremental Conductance + Integral Regulator'  technique  ==
  V_PV : Inport
  I_PV : Inport  Port=2
  Add : Sum  Inputs=+-
  Deblock MPPT : Step  Time=0.4  SampleTime=0
  Duty Cycle : Constant  Value=Dinit
  MPPT : Subsystem
  PWM Generator (DC-DC) : powerlib_meascontrol/Pulse & Signal Generators/PWM Generator (DC-DC)  Fsw=fc  Ts=Ts_Power
  Saturation : Saturate  UpperLimit=1  LowerLimit=0
  Pulses : Outport  VectorParamsAs1DForOutWhenUnconnected=off
  tag scope: D=global
  wires:
  V_PV/1 -> MPPT/1(V_PV)
  I_PV/1 -> MPPT/2(I_PV)
  PWM Generator (DC-DC)/1 -> Pulses/1
  Deblock MPPT/1 -> MPPT/3(on/off)
  Saturation/1 -> PWM Generator (DC-DC)/1, [D]
  Add/1 -> Saturation/1  "D"
  MPPT/1(Delta_D) -> Add/2
  Duty Cycle/1 -> Add/1

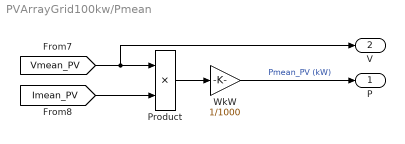
== system PVArrayGrid100kw/Pmean ==
  Product : Product  RndMeth=Zero
  WkW : Gain  Gain=1/1000
  P : Outport  VectorParamsAs1DForOutWhenUnconnected=off
  V : Outport  Port=2  VectorParamsAs1DForOutWhenUnconnected=off
  wires:
  [Vmean_PV] -> Product/1, V/1
  Product/1 -> WkW/1
  [Imean_PV] -> Product/2
  WkW/1 -> P/1  "Pmean_PV (kW)"

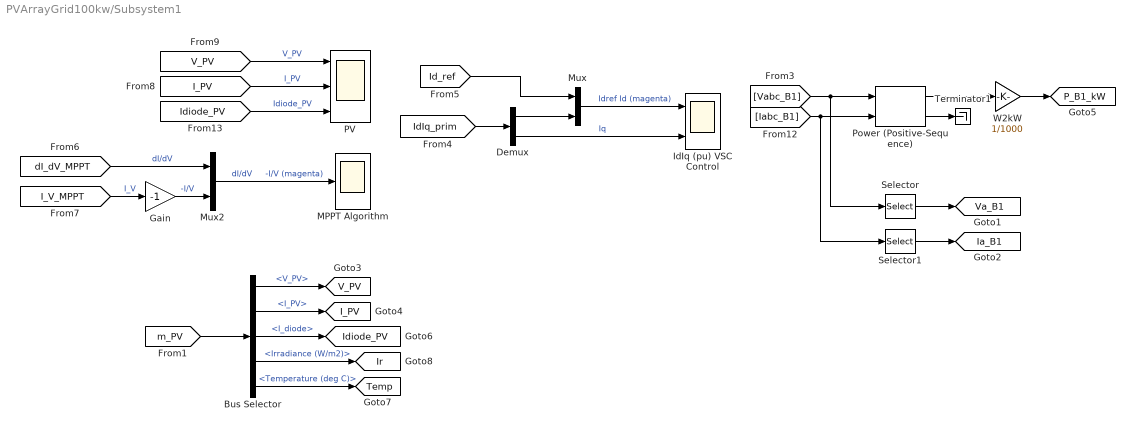
== system PVArrayGrid100kw/Subsystem1 ==
  Bus Selector : BusSelector  OutputSignals=V_PV,I_PV,I_diode,Irradiance (W/m2),Temperature (deg C)
  Demux : Demux  Outputs=2
  Gain : Gain  Gain=-1
  IdIq (pu) VSC Control : Scope  NumInputPorts=2
  MPPT Algorithm : Scope
  Mux : Mux  Inputs=2
  Mux2 : Mux  Inputs=2
  PV : Scope  NumInputPorts=3
  Power (Positive-Sequence) : powerlib_meascontrol/Measurements/Power (Positive-Sequence)  Freq=60  Vinit=[0, 0]  Iinit=[0, 0]  Ts=Ts_Control
  Selector : Selector  InputPortWidth=3  IndexOptions=Index vector (dialog)  Indices=[1]  OutputSizes=1
  Selector1 : Selector  InputPortWidth=3  IndexOptions=Index vector (dialog)  Indices=[1]  OutputSizes=1
  Terminator1 : Terminator
  W2kW : Gain  Gain=1/1000
  tag scope: I_PV=global, Ia_B1=global, Idiode_PV=global, Ir=global, P_B1_kW=global, Temp=global, V_PV=global, Va_B1=global
  wires:
  [Vabc_B1] -> Power (Positive-Sequence)/1, Selector/1
  [Iabc_B1] -> Power (Positive-Sequence)/2, Selector1/1
  Power (Positive-Sequence)/1 -> W2kW/1
  [I_V_MPPT] -> Gain/1  "I_V"
  [IdIq_prim] -> Demux/1
  [Id_ref] -> Mux/1
  Demux/1 -> Mux/2
  Mux/1 -> IdIq (pu) VSC Control/1  "Idref Id (magenta)"
  Demux/2 -> IdIq (pu) VSC Control/2  "Iq"
  Selector/1 -> [Va_B1]
  Selector1/1 -> [Ia_B1]
  [V_PV] -> PV/1  "V_PV"
  [I_PV] -> PV/2  "I_PV"
  [Idiode_PV] -> PV/3  "Idiode_PV"
  [dI_dV_MPPT] -> Mux2/1  "dI/dV"
  Gain/1 -> Mux2/2  "-I/V"
  Mux2/1 -> MPPT Algorithm/1  "dI/dV     -I/V (magenta)"
  W2kW/1 -> [P_B1_kW]
  [m_PV] -> Bus Selector/1
  Bus Selector/1 -> [V_PV]  "<V_PV>"
  Bus Selector/2 -> [I_PV]  "<I_PV>"
  Bus Selector/4 -> [Ir]  "<Irradiance (W/m2)>"
  Bus Selector/3 -> [Idiode_PV]  "<I_diode>"
  Bus Selector/5 -> [Temp]  "<Temperature (deg C)>"
  Power (Positive-Sequence)/2 -> Terminator1/1

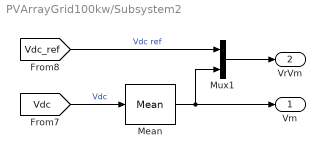
== system PVArrayGrid100kw/Subsystem2 ==
  Mean : powerlib_meascontrol/Measurements/Mean  Freq=60  Vinit=0  Ts=Ts_Control
  Mux1 : Mux  Inputs=2
  Vm : Outport  VectorParamsAs1DForOutWhenUnconnected=off
  VrVm : Outport  Port=2  VectorParamsAs1DForOutWhenUnconnected=off
  wires:
  [Vdc_ref] -> Mux1/1  "Vdc ref"
  [Vdc] -> Mean/1  "Vdc"
  Mux1/1 -> VrVm/1
  Mean/1 -> Mux1/2, Vm/1

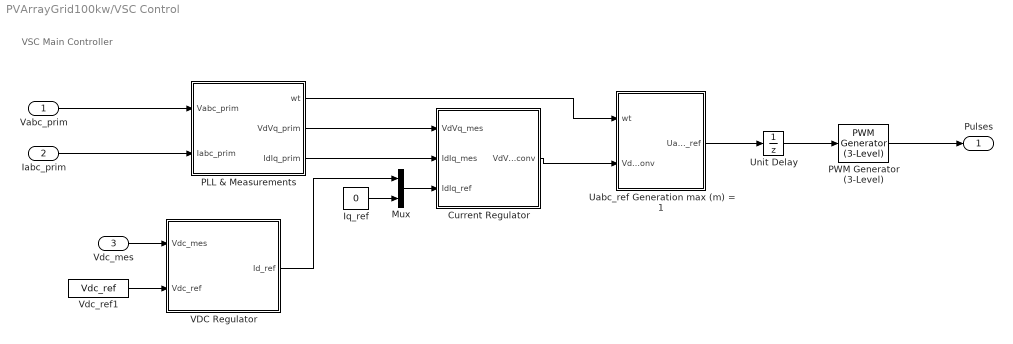
== system PVArrayGrid100kw/VSC Control ==
  note: VSC Main Controller
  Vabc_prim : Inport  PortDimensions=3
  Iabc_prim : Inport  Port=2  PortDimensions=3
  Vdc_mes : Inport  Port=3  PortDimensions=1
  Current Regulator : Subsystem
  Iq_ref : Constant  Value=0
  Mux : Mux  Inputs=2
  PLL & Measurements : Subsystem
  PWM Generator (3-Level) : powerlib_meascontrol/Pulse & Signal Generators/PWM Generator (3-Level)  ModulatorType=Three-phase bridge (12 pulses)  ModulatorMode=Unsynchronized  nF=27  Fc=33*60  ModulatingSignals=off  m=0.8  Freq=60  Phase=0  Ts=Ts_Power
  Uabc_ref Generation max (m) = 1 : Subsystem
  Unit Delay : UnitDelay  SampleTime=Ts_Control  HasFrameUpgradeWarning=on
  VDC Regulator : Subsystem
  Vdc_ref1 : Constant  Value=Vdc_ref
  Pulses : Outport  VectorParamsAs1DForOutWhenUnconnected=off
  wires:
  VDC Regulator/1(Id_ref) -> Mux/1
  PLL & Measurements/1(wt) -> Uabc_ref Generation max (m) = 1/1(wt)
  Current Regulator/1(VdVq_conv) -> Uabc_ref Generation max (m) = 1/2(VdVq_conv)
  Iq_ref/1 -> Mux/2
  Mux/1 -> Current Regulator/3(IdIq_ref)
  PLL & Measurements/3(IdIq_prim) -> Current Regulator/2(IdIq_mes)
  PLL & Measurements/2(VdVq_prim) -> Current Regulator/1(VdVq_mes)
  Vdc_mes/1 -> VDC Regulator/1(Vdc_mes)
  Vabc_prim/1 -> PLL & Measurements/1(Vabc_prim)
  Iabc_prim/1 -> PLL & Measurements/2(Iabc_prim)
  Unit Delay/1 -> PWM Generator (3-Level)/1
  PWM Generator (3-Level)/1 -> Pulses/1
  Uabc_ref Generation max (m) = 1/1(Uabc_ref) -> Unit Delay/1
  Vdc_ref1/1 -> VDC Regulator/2(Vdc_ref)

== system PVArrayGrid100kw/info ==

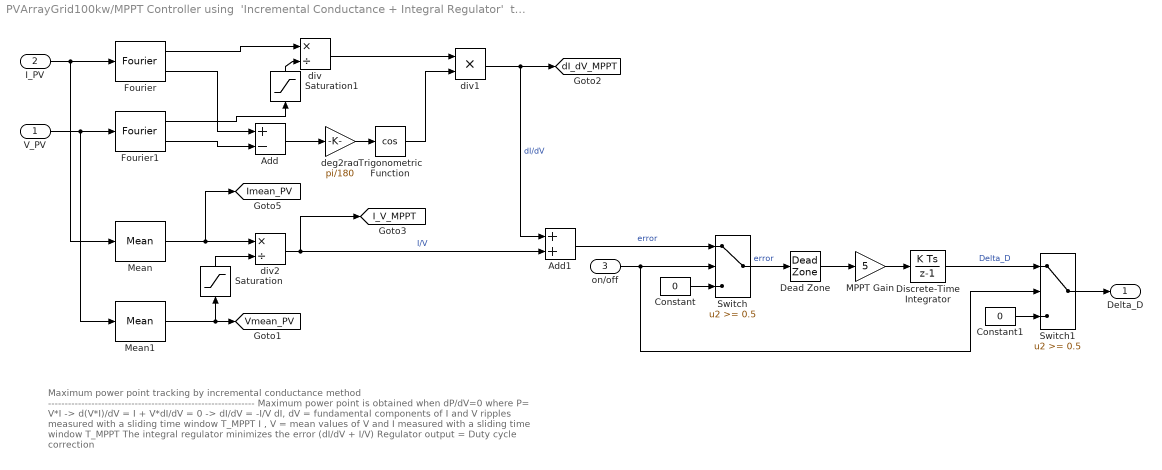
== system PVArrayGrid100kw/MPPT Controller using  'Incremental Conductance + Integral Regulator'  technique /MPPT ==
  note: Maximum power point tracking by incremental conductance method
      | --------------------------------------------------------------
      | Maximum power point is obtained when dP/dV=0  where P= V*I
      | -> d(V*I)/dV = I + V*dI/dV = 0
      | -> dI/dV = -I/V
      |
      | dI, dV  = fundamental components of I and V ripples measured with a sliding time window T_MPPT
      | I , V   = mean values of V and I measured with a sliding time window T_MPPT
      |
      | The integral regulator minimizes the error (dI/dV + I/V)
      | Regulator output = Duty cycle correction
  V_PV : Inport
  I_PV : Inport  Port=2
  on/off : Inport  Port=3
  Add : Sum  Inputs=+-
  Add1 : Sum
  Constant : Constant  Value=0
  Constant1 : Constant  Value=0
  Dead Zone : DeadZone  LowerValue=-0.05  UpperValue=0.05  SaturateOnIntegerOverflow=on
  Discrete-Time Integrator : DiscreteIntegrator  SampleTime=Ts_Control  LimitOutput=on  UpperSaturationLimit=1  LowerSaturationLimit=-1  ICPrevOutput=DiscIntNeverNeededParam  ICPrevScaledInput=DiscIntNeverNeededParam
  Fourier : powerlib_meascontrol/Measurements/Fourier  Freq=1/T_MPPT  n=1  InInit=[0, 0]  Ts=Ts_Control
  Fourier1 : powerlib_meascontrol/Measurements/Fourier  Freq=1/T_MPPT  n=1  InInit=[0, 0]  Ts=Ts_Control
  MPPT Gain : Gain  Gain=5
  Mean : powerlib_meascontrol/Measurements/Mean  Freq=1/T_MPPT  Vinit=0  Ts=Ts_Control
  Mean1 : powerlib_meascontrol/Measurements/Mean  Freq=1/T_MPPT  Vinit=0  Ts=Ts_Control
  Saturation : Saturate  UpperLimit=inf  LowerLimit=eps
  Saturation1 : Saturate  UpperLimit=inf  LowerLimit=eps
  Switch : Switch  Threshold=0.5
  Switch1 : Switch  Threshold=0.5
  Trigonometric Function : Trigonometry  Operator=cos
  deg2rad : Gain  Gain=pi/180
  div : Product  Inputs=*/  RndMeth=Zero
  div1 : Product  Inputs=**  RndMeth=Zero
  div2 : Product  Inputs=*/  RndMeth=Zero
  Delta_D : Outport  VectorParamsAs1DForOutWhenUnconnected=off
  tag scope: I_V_MPPT=global, Imean_PV=global, Vmean_PV=global, dI_dV_MPPT=global
  wires:
  Dead Zone/1 -> MPPT Gain/1
  Switch/1 -> Dead Zone/1  "error"
  Saturation1/1 -> div/2
  Saturation/1 -> div2/2
  Switch1/1 -> Delta_D/1
  on/off/1 -> Switch/2, Switch1/2
  Constant1/1 -> Switch1/3
  Discrete-Time Integrator/1 -> Switch1/1  "Delta_D"
  Constant/1 -> Switch/3
  MPPT Gain/1 -> Discrete-Time Integrator/1
  Add1/1 -> Switch/1  "error"
  div2/1 -> Add1/2, [I_V_MPPT]  "I/V"
  Mean1/1 -> Saturation/1, [Vmean_PV]
  Mean/1 -> div2/1, [Imean_PV]
  div1/1 -> Add1/1, [dI_dV_MPPT]  "dI/dV"
  Trigonometric Function/1 -> div1/2
  div/1 -> div1/1
  deg2rad/1 -> Trigonometric Function/1
  Add/1 -> deg2rad/1
  Fourier1/1 -> Saturation1/1
  Fourier1/2 -> Add/2
  Fourier/2 -> Add/1
  V_PV/1 -> Mean1/1, Fourier1/1
  I_PV/1 -> Mean/1, Fourier/1
  Fourier/1 -> div/1

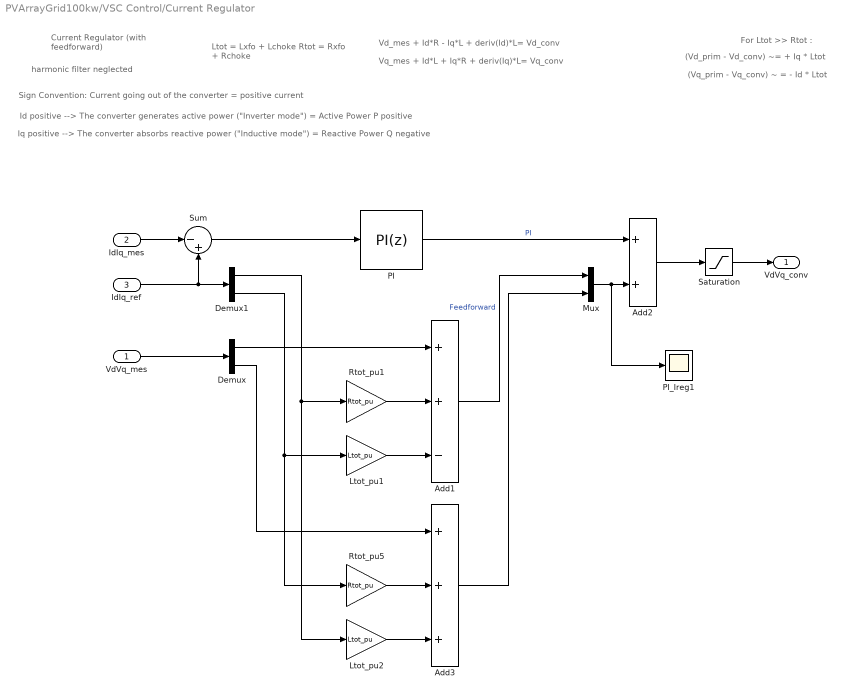
== system PVArrayGrid100kw/VSC Control/Current Regulator ==
  note: harmonic filter neglected
  note: Vd_mes + Id*R - Iq*L + deriv(Id)*L= Vd_conv
  note: Vq_mes + Id*L + Iq*R + deriv(Iq)*L= Vq_conv
  note: Current Regulator
      | (with feedforward)
  note: Sign Convention: Current going out of the converter = positive current
  note: Iq positive --> The converter absorbs reactive power ("Inductive mode") = Reactive Power Q negative
  note: Id positive --> The converter generates active power ("Inverter mode") = Active Power P positive
  note: Ltot = Lxfo + Lchoke
      | Rtot = Rxfo + Rchoke
  note: (Vd_prim - Vd_conv) ~= + Iq * Ltot
  note: (Vq_prim - Vq_conv) ~ = - Id * Ltot
  note: For Ltot >> Rtot :
  VdVq_mes : Inport  PortDimensions=2
  IdIq_mes : Inport  Port=2  PortDimensions=2
  IdIq_ref : Inport  Port=3  PortDimensions=2
  Add1 : Sum  Inputs=++-
  Add2 : Sum
  Add3 : Sum  Inputs=+++
  Demux : Demux  Outputs=2
  Demux1 : Demux  Outputs=2
  Ltot_pu1 : Gain  Gain=Ltot_pu  SaturateOnIntegerOverflow=on  OutDataTypeStr=Inherit: Same as input  ParamDataTypeStr=Inherit: Same as input
  Ltot_pu2 : Gain  Gain=Ltot_pu  SaturateOnIntegerOverflow=on  OutDataTypeStr=Inherit: Same as input  ParamDataTypeStr=Inherit: Same as input
  Mux : Mux  Inputs=2
  PI : simulink/Continuous/PID Controller  Controller=PI  Form=Parallel  TimeDomain=Discrete-time  SampleTime=Ts  IntegratorMethod=Forward Euler  ControllerParametersSource=internal  P=Kp_Ireg  I=Ki_Ireg  D=0  N=100  UseFilter=on  TunerSelectOption=Transfer Function Based (PID Tuner App)  InitialConditionSource=internal  InitialConditionForIntegrator=0  InitialConditionForFilter=0  DifferentiatorICPrevScaledInput=0  ExternalReset=none  TrackingMode=off  Kt=1  LimitOutput=on  UpperSaturationLimit=2  LowerSaturationLimit=-2  LinearizeAsGain=off  AntiWindupMode=none  Kb=1  POutMin=[]  POutMax=[]  IOutMin=[]  IOutMax=[]  DOutMin=[]  DOutMax=[]  NOutMin=[]  NOutMax=[]  SumOutMin=[]  SumOutMax=[]  SaturationOutMin=[]  SaturationOutMax=[]  PParamMin=[]  PParamMax=[]  IParamMin=[]  IParamMax=[]  DParamMin=[]  DParamMax=[]  NParamMin=[]  NParamMax=[]  KbParamMin=[]  KbParamMax=[]  KtParamMin=[]  KtParamMax=[]  KbOutMin=[]  KbOutMax=[]  KtOutMin=[]  KtOutMax=[]  IntegratorOutMin=[]  IntegratorOutMax=[]  FilterOutMin=[]  FilterOutMax=[]  SumI1OutMin=[]  SumI1OutMax=[]  SumI2OutMin=[]  SumI2OutMax=[]  SumI3OutMin=[]  SumI3OutMax=[]  SumI4OutMin=[]  SumI4OutMax=[]  SumDOutMin=[]  SumDOutMax=[]  DifferentiatorOutMin=[]  DifferentiatorOutMax=[]  FilterDiffOutCoefMin=[]  FilterDiffOutCoefMax=[]  ReciprocalOutMin=[]  ReciprocalOutMax=[]  SumDenOutMin=[]  SumDenOutMax=[]  SumNumOutMin=[]  SumNumOutMax=[]  DivideOutMin=[]  DivideOutMax=[]  IntegratorContinuousStateAttributes=''  IntegratorStateMustResolveToSignalObject=off  IntegratorRTWStateStorageClass=Auto  FilterContinuousStateAttributes=''  FilterStateMustResolveToSignalObject=off  FilterRTWStateStorageClass=Auto  ParallelPVariant=InternalParameters  IdealPVariant=Disabled  IVariant=InternalParameters  DVariant=Disabled  IntegratorVariant=Discrete  SatVariant=Enabled  AWVariant=Passthrough  PCopyVariant=Disabled  TRVariant=Disabled  FdbkBlocksVariant=Forward  IdealPFdbkVariant=Disabled  SatFdbkVariant=Disabled  DerivativeFilterVariant=Disabled  NVariant=Disabled  NCopyVariant=Disabled_SignalSpec  FilterICVariant=Disabled  IntegratorICVariant=InternalICs  ExternalResetVariant=Disabled  TRSumVariant=Passthrough  SumFdbkVariant=Disabled  SumVariant=Sum_PI
  PI_Ireg1 : Scope
  Rtot_pu1 : Gain  Gain=Rtot_pu  SaturateOnIntegerOverflow=on  OutDataTypeStr=Inherit: Same as input  ParamDataTypeStr=Inherit: Same as input
  Rtot_pu5 : Gain  Gain=Rtot_pu  SaturateOnIntegerOverflow=on  OutDataTypeStr=Inherit: Same as input  ParamDataTypeStr=Inherit: Same as input
  Saturation : Saturate  UpperLimit=2  LowerLimit=-2
  Sum : Sum  Inputs=|-+
  VdVq_conv : Outport  VectorParamsAs1DForOutWhenUnconnected=off
  wires:
  Mux/1 -> PI_Ireg1/1, Add2/2
  PI/1 -> Add2/1  "PI"
  Sum/1 -> PI/1
  IdIq_ref/1 -> Sum/2, Demux1/1
  IdIq_mes/1 -> Sum/1
  Add2/1 -> Saturation/1
  Saturation/1 -> VdVq_conv/1
  VdVq_mes/1 -> Demux/1
  Demux/1 -> Add1/1
  Rtot_pu1/1 -> Add1/2
  Demux1/1 -> Rtot_pu1/1, Ltot_pu2/1
  Ltot_pu1/1 -> Add1/3
  Demux1/2 -> Ltot_pu1/1, Rtot_pu5/1
  Rtot_pu5/1 -> Add3/2
  Ltot_pu2/1 -> Add3/3
  Add1/1 -> Mux/1  "Feedforward"
  Demux/2 -> Add3/1
  Add3/1 -> Mux/2
